simulink model "test_sendrcv"  (R2021a)
settings: Solver=FixedStepDiscrete  StartTime=0.0  StopTime=100  FixedStep=0.05  RelTol=1e-3  EnableMultiTasking=on
values from neighbouring files (symbols this model uses):
  c1 = 5.0    [rostest_testsendrcv.sldd]
  KPP_goodDisFrontLen_mm = 50.0    [rostest_testsendrcv.sldd]
  KPP_safeDisRearLen_mm = 50.0    [rostest_testsendrcv.sldd]
  KPP_safeDisSideWidth_mm = 20.0    [rostest_testsendrcv.sldd]
  map2d = 7.0 44.0 18.0 3.0 96.0 44.0 97.0 77.0 1.0 69.0 71.0 65.0 56.0 22.0 78.0 23.0 38.0 90.0 86.0 41.0 32.0 61.0 92.0 91.0 60.0 34.0 86.0 45.0 91.0 4.0 54.0 72.0 18.0 34.0 19.0 33.0 41.0 55.0 5.0 56.0 28.0 25.0 25.0 16.0 96.0 94.0 82.0 73.0 18.0 37.0 19.0 1.0 32.0 70.0 63.0 55.0 44.0 29.0 51.0 77.0 77.0 58.0 75.0 65.0 13.0 51.0 35.0 10.0 15.0 20.0 68.0 44.0 70.0 26.0 1.0 54.0 28.0 95.0 91.0 40.0 3.0 68.    [rostest_testsendrcv.sldd]
  map2d_x : value not decoded    [rostest_testsendrcv.sldd]
  map2d_y : value not decoded    [rostest_testsendrcv.sldd]
  POLYGON_MAXITER = 4.0    [rostest_testsendrcv.sldd]
  polygoni_x_ovrdflg = 0.0    [rostest_testsendrcv.sldd]
  polygoni_x_ovrdval = 0.21    [rostest_testsendrcv.sldd]
  polygonj_x_ovrdflg = 0.0    [rostest_testsendrcv.sldd]
  polygonj_x_ovrdval = 0.32    [rostest_testsendrcv.sldd]
  pt_x_ovrdflg = 0.0    [rostest_testsendrcv.sldd]
  pt_x_ovrdval = 0.1    [rostest_testsendrcv.sldd]
  x_input : value not decoded    [rostest_testsendrcv.sldd]
  x_output : value not decoded    [rostest_testsendrcv.sldd]
libraries: coros_protocol_lib x1
settings Model: DataDictionary=rostest_testsendrcv.sldd  SimulationMode=external  Creator=xuliangliang  LastModifiedBy=MyPC
settings OptimizationCC: EnhancedBackFolding=on  PassReuseOutputArgsAs=Individual arguments  ZeroExternalMemoryAtStartup=off  ZeroInternalMemoryAtStartup=off  MaxStackSize=64  OptimizeBlockOrder=speed  DifferentSizesBufferReuse=on  OptimizationCustomize=off  EfficientTunableParamExpr=on
settings DebuggingCC: ParameterTunabilityLossMsg=error
settings HardwareCC: ProdBitPerLong=64  ProdHWDeviceType=AMD->x86-64 (Linux 64)
settings SFSimCC: MATLABDynamicMemAlloc=off  SimTargetLang=C++
settings RTWCC: SystemTargetFile=ert.tlc  HardwareBoard=Robot Operating System (ROS)  TLCOptions="-aInlineSetEventsForThisBaseRateFcn=TLC_FALSE -aSuppressMultiTaskScheduler=TLC_FALSE  -aRateBasedStepFcn=0"  TemplateMakefile=ert_default_tmf  PostCodeGenCommand=postcode_process(buildInfo)  RetainRTWFile=on  RTWUseSimCustomCode=on  Toolchain=Catkin  TargetLang=C++
settings CodeAppCC: ForceParamTrailComments=on  IgnoreCustomStorageClasses=off  OperatorAnnotations=on  SimulinkDataObjDesc=on  SFDataObjDesc=on  InsertBlockDesc=on

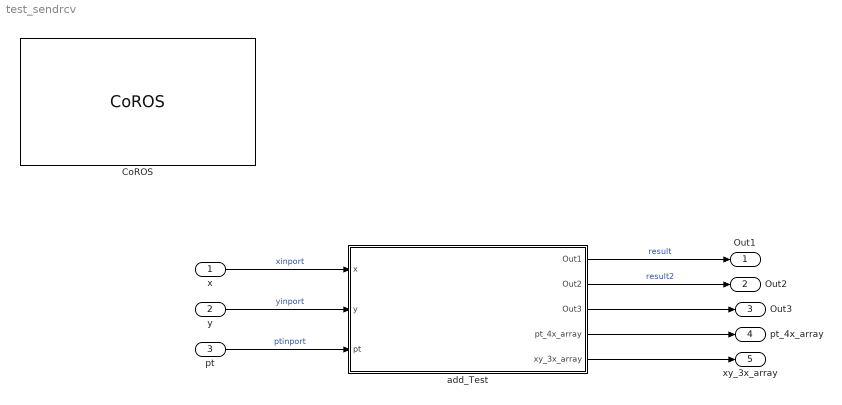
== system test_sendrcv ==
  x : Inport  OutDataTypeStr=single
  y : Inport  Port=2  OutDataTypeStr=single
  pt : Inport  Port=3  OutDataTypeStr=Bus: point_t
  CoROS : coros_protocol_lib/CoROS  SystemSampleTime=-1  VariantActivationTime=update diagram  Latency=0  AutoFrameSizeCalculation=off
      link override CoROS_QueueTx/TX/Bus creator: OutDataTypeStr=Bus: SL_Bus_test_sendrcv_coros_msgs_resppacket
  add_Test : Subsystem  TreatAsAtomicUnit=on
  Out1 : Outport  OutDataTypeStr=single
  Out2 : Outport  Port=2  OutDataTypeStr=single
  Out3 : Outport  Port=3
  pt_4x_array : Outport  Port=4
  xy_3x_array : Outport  Port=5
  wires:
  add_Test/2(Out2) -> Out2/1  "result2"
  x/1 -> add_Test/1(x)  "xinport"
  y/1 -> add_Test/2(y)  "yinport"
  add_Test/1(Out1) -> Out1/1  "result"
  pt/1 -> add_Test/3(pt)  "ptinport"
  add_Test/3(Out3) -> Out3/1
  add_Test/4(pt_4x_array) -> pt_4x_array/1
  add_Test/5(xy_3x_array) -> xy_3x_array/1

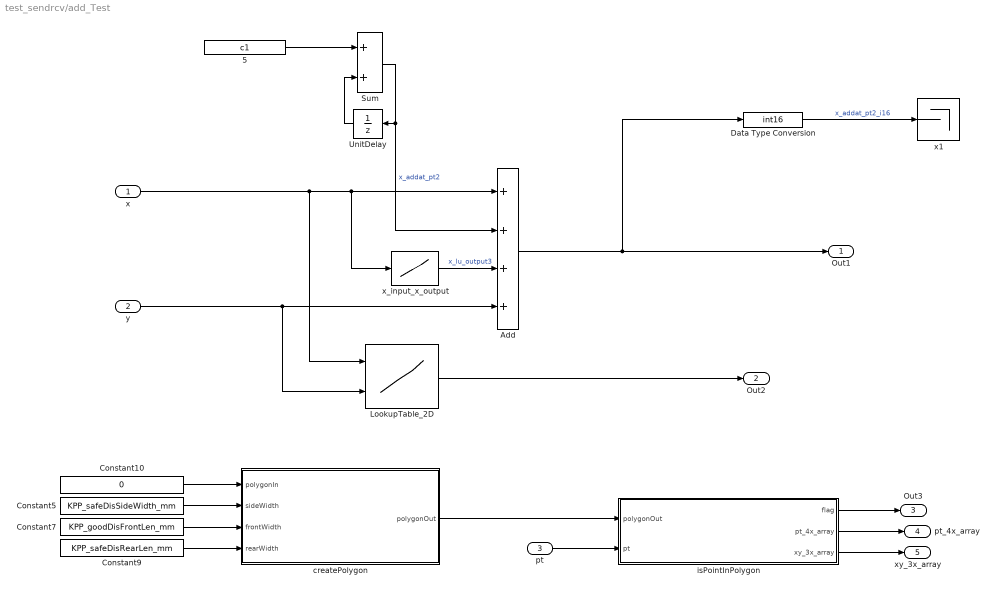
== system test_sendrcv/add_Test ==
  x : Inport
  y : Inport  Port=2
  pt : Inport  Port=3
  5 : Constant  Value=c1
  Add : Sum  Inputs=++++
  Constant10 : Constant  Value=0  OutDataTypeStr=Bus: Polygon_t
  Constant5 : Constant  Value=KPP_safeDisSideWidth_mm  OutDataTypeStr=single
  Constant7 : Constant  Value=KPP_goodDisFrontLen_mm  OutDataTypeStr=single
  Constant9 : Constant  Value=KPP_safeDisRearLen_mm  OutDataTypeStr=single
  Data Type Conversion : DataTypeConversion  OutDataTypeStr=int16  SaturateOnIntegerOverflow=on  RndMeth=Zero
  LookupTable_2D : Lookup_n-D  BreakpointsForDimension1=map2d_y  BreakpointsForDimension2=map2d_x  Table=map2d  TableDataTypeStr=Inherit: Inherit from 'Table data'  ExtrapMethod=Clip  UseLastTableValue=on  InternalRulePriority=Speed  OutDataTypeStr=Inherit: Inherit from 'Table data'  RndMeth=Zero
      settings: InputPortMap=u0,u1
      settings: AttributesFormatString=|
      | <X Axis = %<BreakpointsForDimension1>>
      | <Y Axis = %<BreakpointsForDimension2>>
      | <Table = %<Table>>
      | <InterpMethod = %<InterpMethod>; ExtrapMethod = %<ExtrapMethod>; UseLastTableValue: %<UseLastTableValue>>
  Sum : Sum
  UnitDelay : UnitDelay  SampleTime=-1
      settings: AttributesFormatString=Init: %<X0>
  createPolygon : MATLAB Function  TreatAsAtomicUnit=on
  isPointInPolygon : Subsystem
      mask Display: disp('isPointInPolygon')
  x1 : Terminator
  x_input_x_output : Lookup_n-D  NumberOfTableDimensions=1  BreakpointsForDimension1=x_input  Table=x_output  InternalRulePriority=Speed  RndMeth=Simplest  InputSameDT=on
  Out1 : Outport
  Out2 : Outport  Port=2
  Out3 : Outport  Port=3
  pt_4x_array : Outport  Port=4
  xy_3x_array : Outport  Port=5
  wires:
  x/1 -> LookupTable_2D/1, x_input_x_output/1, Add/1
  y/1 -> LookupTable_2D/2, Add/4
  x_input_x_output/1 -> Add/3  "x_lu_output3"
  LookupTable_2D/1 -> Out2/1
  Constant9/1 -> createPolygon/4(rearWidth)
  Constant7/1 -> createPolygon/3(frontWidth)
  Constant5/1 -> createPolygon/2(sideWidth)
  Constant10/1 -> createPolygon/1(polygonIn)
  createPolygon/1(polygonOut) -> isPointInPolygon/1(polygonOut)
  pt/1 -> isPointInPolygon/2(pt)
  isPointInPolygon/1(flag) -> Out3/1
  isPointInPolygon/2(pt_4x_array) -> pt_4x_array/1
  isPointInPolygon/3(xy_3x_array) -> xy_3x_array/1
  5/1 -> Sum/1
  Sum/1 -> Add/2, UnitDelay/1  "x_addat_pt2"
  UnitDelay/1 -> Sum/2
  Add/1 -> Out1/1, Data Type Conversion/1
  Data Type Conversion/1 -> x1/1  "x_addat_pt2_i16"

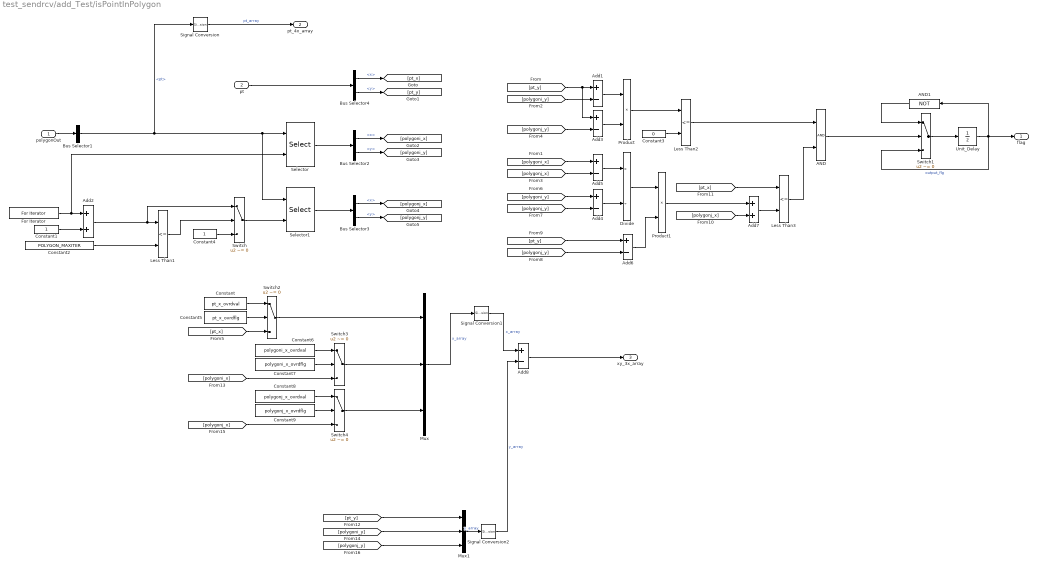
== system test_sendrcv/add_Test/isPointInPolygon ==
  polygonOut : Inport
  pt : Inport  Port=2
  AND : Logic  AllPortsSameDT=off  OutDataTypeStr=boolean
  AND1 : Logic  Operator=NOT  AllPortsSameDT=off  OutDataTypeStr=boolean
  Add{1,3..6,8} (6 alike) : Sum  Inputs=+-
  Add2 : Sum
  Add7 : Sum
  Bus Selector1 : BusSelector  OutputSignals=pt
  Bus Selector2 : BusSelector  OutputSignals=x,y
  Bus Selector3 : BusSelector  OutputSignals=x,y
  Bus Selector4 : BusSelector  OutputSignals=x,y
  Constant : Constant  Value=pt_x_ovrdval
  Constant1 : Constant  OutDataTypeStr=int32
  Constant2 : Constant  Value=POLYGON_MAXITER  OutDataTypeStr=int32
  Constant3 : Constant  Value=0  OutDataTypeStr=single
  Constant4 : Constant  OutDataTypeStr=int32
  Constant5 : Constant  Value=pt_x_ovrdflg  OutDataTypeStr=boolean
  Constant6 : Constant  Value=polygoni_x_ovrdval
  Constant7 : Constant  Value=polygoni_x_ovrdflg  OutDataTypeStr=boolean
  Constant8 : Constant  Value=polygonj_x_ovrdval
  Constant9 : Constant  Value=polygonj_x_ovrdflg  OutDataTypeStr=boolean
  Divide : Product  Inputs=*/
  For Iterator : ForIterator  ResetStates=reset  IterationLimit=POLYGON_MAXITER
  Less Than1 : RelationalOperator  Operator=<=  OutDataTypeStr=boolean  RndMeth=Simplest
  Less Than2 : RelationalOperator  Operator=<=  OutDataTypeStr=boolean  RndMeth=Simplest
  Less Than3 : RelationalOperator  Operator=<=  OutDataTypeStr=boolean  RndMeth=Simplest
  Mux : Mux  Inputs=3
  Mux1 : Mux  Inputs=3
  Product : Product
  Product1 : Product
  Selector : Selector  IndexOptions=Starting index (port)  Indices=[1 3]  OutputSizes=1
  Selector1 : Selector  IndexOptions=Starting index (port)  Indices=[1 3]  OutputSizes=1
  Signal Conversion : SignalConversion  OverrideOpt=off
  Signal Conversion1 : SignalConversion  OverrideOpt=off
  Signal Conversion2 : SignalConversion  OverrideOpt=off
  Switch : Switch  Criteria=u2 ~= 0  RndMeth=Zero
      settings: AttributesFormatString=<%<Criteria>>
  Switch1 : Switch  Criteria=u2 ~= 0  RndMeth=Zero
      settings: AttributesFormatString=<%<Criteria>>
  Switch2 : Switch  Criteria=u2 ~= 0  SaturateOnIntegerOverflow=on  InputSameDT=on
  Switch3 : Switch  Criteria=u2 ~= 0  SaturateOnIntegerOverflow=on  InputSameDT=on
  Switch4 : Switch  Criteria=u2 ~= 0  SaturateOnIntegerOverflow=on  InputSameDT=on
  Unit_Delay : UnitDelay  InitialCondition=false  SampleTime=-1  HasFrameUpgradeWarning=on
      settings: AttributesFormatString=|
      | <init value = %<InitialCondition>>
      | <sample time = %<SampleTime>>
  flag : Outport
  pt_4x_array : Outport  Port=2
  xy_3x_array : Outport  Port=3
  wires:
  Constant1/1 -> Add2/2
  polygonOut/1 -> Bus Selector1/1
  pt/1 -> Bus Selector4/1
  Constant2/1 -> Less Than1/2
  Constant4/1 -> Switch/3
  Less Than1/1 -> Switch/2
  Add2/1 -> Less Than1/1, Switch/1
  Bus Selector1/1 -> Selector/1, Selector1/1, Signal Conversion/1  "<pt>"
  Switch/1 -> Selector1/2
  For Iterator/1 -> Selector/2, Add2/1
  Selector/1 -> Bus Selector2/1
  Selector1/1 -> Bus Selector3/1
  Add1/1 -> Product/1
  Add3/1 -> Product/2
  Product/1 -> Less Than2/1
  Constant3/1 -> Less Than2/2
  Bus Selector4/1 -> [pt_x]  "<x>"
  Bus Selector4/2 -> [pt_y]  "<y>"
  Bus Selector2/1 -> [polygoni_x]  "<x>"
  Bus Selector2/2 -> [polygoni_y]  "<y>"
  Bus Selector3/1 -> [polygonj_x]  "<x>"
  Bus Selector3/2 -> [polygonj_y]  "<y>"
  [pt_y] -> Add3/1, Add1/1
  [polygoni_y] -> Add1/2
  [polygonj_y] -> Add3/2
  [polygoni_y] -> Add4/1
  [polygonj_y] -> Add4/2
  [polygoni_x] -> Add5/1
  [polygonj_x] -> Add5/2
  Add5/1 -> Divide/1
  Add4/1 -> Divide/2
  Divide/1 -> Product1/1
  Add6/1 -> Product1/2
  [polygonj_y] -> Add6/2
  [pt_y] -> Add6/1
  Product1/1 -> Add7/1
  [polygonj_x] -> Add7/2
  Add7/1 -> Less Than3/2
  [pt_x] -> Less Than3/1
  Less Than2/1 -> AND/1
  Less Than3/1 -> AND/2
  AND/1 -> Switch1/2
  Switch1/1 -> Unit_Delay/1
  Unit_Delay/1 -> Switch1/3, flag/1, AND1/1  "output_flg"
  AND1/1 -> Switch1/1
  Signal Conversion/1 -> pt_4x_array/1  "pt_array"
  [polygonj_y] -> Mux1/3
  [polygoni_y] -> Mux1/2
  [pt_y] -> Mux1/1
  Add8/1 -> xy_3x_array/1
  Mux/1 -> Signal Conversion1/1  "x_array"
  Signal Conversion1/1 -> Add8/1  "x_array"
  Mux1/1 -> Signal Conversion2/1  "y_array"
  Signal Conversion2/1 -> Add8/2  "y_array"
  [pt_x] -> Switch2/3
  Switch2/1 -> Mux/1
  Constant/1 -> Switch2/1
  Constant5/1 -> Switch2/2
  [polygoni_x] -> Switch3/3
  Switch3/1 -> Mux/2
  Constant6/1 -> Switch3/1
  Constant7/1 -> Switch3/2
  [polygonj_x] -> Switch4/3
  Switch4/1 -> Mux/3
  Constant8/1 -> Switch4/1
  Constant9/1 -> Switch4/2

== matlab function test_sendrcv/add_Test/createPolygon ==
  data: polygonIn input Bus: Polygon_t; polygonOut output Bus: Polygon_t; sideWidth input single; frontWidth input single; rearWidth input single
function polygonOut = createPolygon(polygonIn, sideWidth, frontWidth, rearWidth)
    polygonOut = polygonIn;
    polygonOut.ptNum = int32(4);
    polygonOut.pt(1).x = - CAR.RearOH - rearWidth;
    polygonOut.pt(1).y = - CAR.HalfWidth - sideWidth;
    polygonOut.pt(2).x =   CAR.FrontOH + CAR.AxisLen + frontWidth;
    polygonOut.pt(2).y = - CAR.HalfWidth - sideWidth;
    polygonOut.pt(3).x =   CAR.FrontOH + CAR.AxisLen + frontWidth;
    polygonOut.pt(3).y =   CAR.HalfWidth + sideWidth;
    polygonOut.pt(4).x = - CAR.RearOH - rearWidth;
    polygonOut.pt(4).y =   CAR.HalfWidth + sideWidth;
end
